simulink library "exprofilelib"  (Simulink 7.6)
settings: Solver=ode45  SolverMode=SingleTasking  StartTime=0.0  StopTime=10.0  RelTol=1e-3
undefined symbols (not defined in the file or in its folder): T
libraries: simulink x2, exprofilelib x1, simulink_extras x1
settings Model: Creator=The MathWorks Inc.

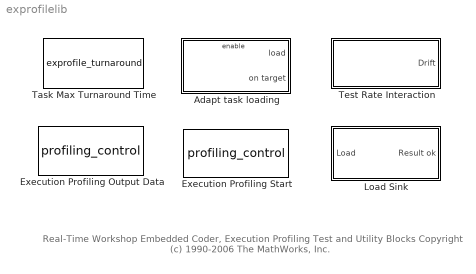
== system exprofilelib ==
  note: Real-Time Workshop Embedded Coder, Execution Profiling Test and Utility Blocks
      | Copyright (c) 1990-2006 The MathWorks, Inc.
  Adapt task loading : Subsystem  mask(Adapt task loading){rateNum=0, target=uint32(1000), adapt=64, t=T}
      mask prompts: rateNum "Rate number:"; target "Target turnaround time in free running timer ticks:"; adapt "Adaptation factor:"; t "Sample time:"
      mask help: Increase the load demand until the task turnaround time reaches the target. The load demand ratchets up at a rate inversely proportional to the adaptation factor.
      mask Display: disp(sprintf(['Target = %d'], double(target)))
  Execution Profiling Output Data : S-Function  FunctionName=profiling_control  Parameters=mode, t  EnableBusSupport=off  mask(Output execution profiling data){t=1}
      mask prompts: t "Sample time"
      mask help: Outputs logged exectution profiling data. The data is output 8 bytes at a time; the active output is set to true while logged data is output.
      mask init:
      | mode = 2; % data output
      mask Display:
      | port_label('output',1,'Data active')
      | port_label('output',2,'Data')
  Execution Profiling Start : S-Function  FunctionName=profiling_control  Parameters=mode, t  EnableBusSupport=off  mask(Start Execution Profiling){}
      mask help: Initiates logging of execution profiling data; this block should typically be placed inside a triggered sub-system.
      mask init:
      | mode = 1; % control input
      | t = -1; % sample time
      mask Display: disp(sprintf('Start\nExecution Profiling'))
  Load Sink : Subsystem  TreatAsAtomicUnit=on  mask(Load Sink){mode=single, t=1}
      mask prompts: t "Sample time:"
      mask help: This block consumes processor time by performing integer or floating point calculations. The larger the value of the load input, the more processor time is consumed.
      mask init:
      | if strcmp(mode,'int16')
      | 	tol_eps = int32(0);
      | 	a = int32(0);
      | elseif strcmp(mode,'single')
      |     tol_eps = single(1.192e-7);
      | 	a = single(3.1415926);
      | else
      | 	error(['Unrecognized value for mode'])
      | end
      settings: RTWSystemCode=Function
      mask StyleString: popup(int16|single),edit
  Task Max Turnaround Time : S-Function  FunctionName=exprofile_turnaround  Parameters=rateNumber, t  EnableBusSupport=off  mask(Task Maximum Turnaround Time){rateNumber=0, t=T*16}
      mask prompts: rateNumber "Rate number:"; t "Sample time:"
      mask help:
      | Outputs the maximum logged turnaround time, in free running timer ticks, for a model timer-based task. A free running timer must have been configured for use with the execution profiling engine. If execution profiling is not enabled, the output is zero.
      |
      | For a model running in multi-tasking mode, the rate number must be in the range 0 to (N-1) where 0 represents the base rate and N is the total number of rates in the model. If the model is running in single tasking mode then the rate number must be zero.
      mask Display: disp(sprintf('Task maximum\nturnaround time'))
  Test Rate Interaction : Subsystem  mask(Test Rate Interaction){t=T}
      mask prompts: t "Faster sample time:"
      mask help:
      | This block contains two tasks, one with the faster sample time, the other running four times slower.
      |
      | Data is transferred continually between the two tasks and tested for consistency. In simulation, the drift output will always be zero. When executing in real-time, the drift output will always be non-zero provided that no sub-rate overruns occur. If sub-rate overruns do occur then data transfer between rates may be delayed causing the drift output to be non-zero.
      mask Display: disp(sprintf('Test rate\n interaction'))

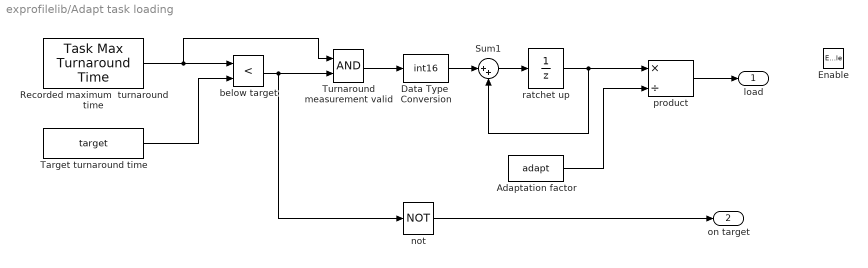
== system exprofilelib/Adapt task loading ==
  Enable : EnablePort
  Adaptation factor : Constant  Value=adapt  OutDataTypeStr=Inherit: Inherit via back propagation
  Data Type  Conversion : DataTypeConversion  OutDataTypeStr=int16  SaturateOnIntegerOverflow=on  RndMeth=Zero
  Recorded maximum  turnaround time : exprofilelib/Task Max Turnaround Time  rateNumber=rateNum  t=t
  Sum1 : Sum  Inputs=|++  InputSameDT=on
  Target turnaround time : Constant  Value=target
  Turnaround measurement valid : Logic  AllPortsSameDT=off  OutDataTypeStr=uint(8)
  below target : RelationalOperator  Operator=<  InputSameDT=on
  not : Logic  Operator=NOT  AllPortsSameDT=off  OutDataTypeStr=uint(8)
  product : Product  Inputs=*/  InputSameDT=on  OutDataTypeStr=Inherit: Same as first input
  ratchet up : UnitDelay  SampleTime=-1
  load : Outport
  on target : Outport  Port=2
  wires:
  not/1 -> on target/1
  Target turnaround time/1 -> below target/2
  product/1 -> load/1
  Recorded maximum  turnaround time/1 -> below target/1, Turnaround measurement valid/1
  Adaptation factor/1 -> product/2
  Data Type  Conversion/1 -> Sum1/1
  ratchet up/1 -> product/1, Sum1/2
  below target/1 -> not/1, Turnaround measurement valid/2
  Sum1/1 -> ratchet up/1
  Turnaround measurement valid/1 -> Data Type  Conversion/1

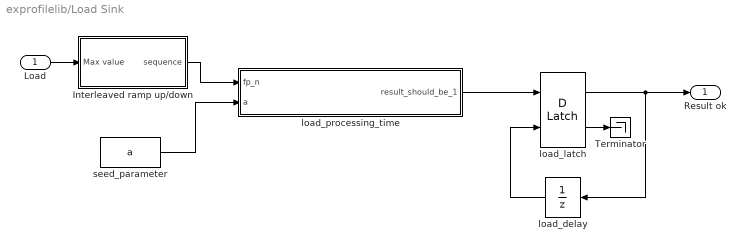
== system exprofilelib/Load Sink ==
  Load : Inport
  Interleaved ramp up/down : Subsystem  mask(Interleaved ramp up/down){t=t}
      mask prompts: t "Sample time:"
  Terminator : Terminator
  load_delay : UnitDelay  X0=1  SampleTime=t
  load_latch : simulink_extras/Flip Flops/D Latch  SystemSampleTime=-1
  load_processing_time : Subsystem
  seed_parameter : Constant  Value=a
  Result ok : Outport
  wires:
  seed_parameter/1 -> load_processing_time/2(a)
  load_processing_time/1(result_should_be_1) -> load_latch/1
  load_latch/1 -> Result ok/1, load_delay/1
  load_delay/1 -> load_latch/2
  load_latch/2 -> Terminator/1
  Interleaved ramp up/down/1(sequence) -> load_processing_time/1(fp_n)
  Load/1 -> Interleaved ramp up/down/1(Max value)

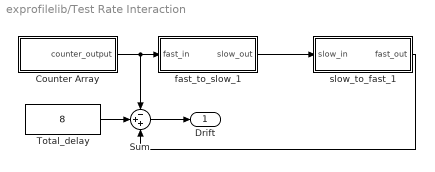
== system exprofilelib/Test Rate Interaction ==
  Counter Array : Subsystem
  Sum : Sum  Inputs=-++  InputSameDT=on
  Total_delay : Constant  Value=8  OutDataTypeStr=Inherit: Inherit via back propagation
  fast_to_slow_1 : Subsystem
  slow_to_fast_1 : Subsystem
  Drift : Outport
  wires:
  fast_to_slow_1/1(slow_out) -> slow_to_fast_1/1(slow_in)
  Counter Array/1(counter_output) -> fast_to_slow_1/1(fast_in), Sum/1
  Total_delay/1 -> Sum/2
  slow_to_fast_1/1(fast_out) -> Sum/3
  Sum/1 -> Drift/1

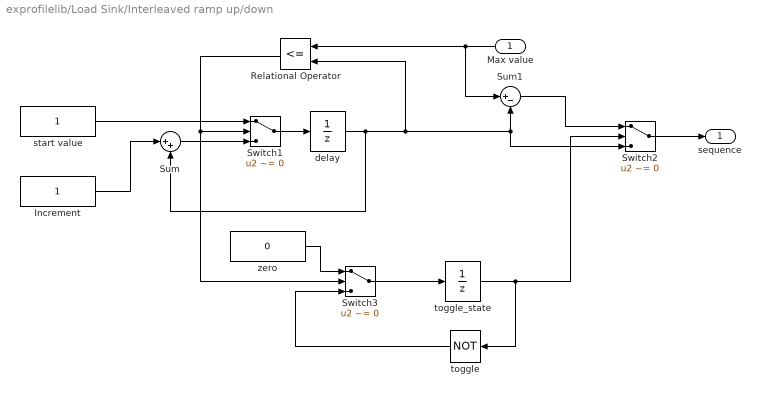
== system exprofilelib/Load Sink/Interleaved ramp up/down ==
  Max value : Inport
  Increment : Constant  OutDataTypeStr=Inherit: Inherit via back propagation
  Relational Operator : RelationalOperator  Operator=<=  InputSameDT=on
  Sum : Sum  Inputs=|++  InputSameDT=on
  Sum1 : Sum  Inputs=|+-
  Switch1 : Switch  Criteria=u2 ~= 0  SaturateOnIntegerOverflow=on  InputSameDT=on
  Switch2 : Switch  Criteria=u2 ~= 0  SaturateOnIntegerOverflow=on
  Switch3 : Switch  Criteria=u2 ~= 0  SaturateOnIntegerOverflow=on  InputSameDT=on
  delay : UnitDelay  X0=1  SampleTime=t
  start value : Constant  OutDataTypeStr=Inherit: Inherit via back propagation
  toggle : Logic  Operator=NOT  AllPortsSameDT=off
  toggle_state : UnitDelay  SampleTime=t
  zero : Constant  Value=0  OutDataTypeStr=Inherit: Inherit via back propagation
  sequence : Outport
  wires:
  zero/1 -> Switch3/1
  Switch3/1 -> toggle_state/1
  toggle/1 -> Switch3/3
  Sum1/1 -> Switch2/1
  toggle_state/1 -> Switch2/2, toggle/1
  start value/1 -> Switch1/1
  Switch2/1 -> sequence/1
  Max value/1 -> Sum1/1, Relational Operator/1
  Relational Operator/1 -> Switch3/2, Switch1/2
  Sum/1 -> Switch1/3
  Switch1/1 -> delay/1
  Increment/1 -> Sum/1
  delay/1 -> Switch2/3, Sum1/2, Relational Operator/2, Sum/2

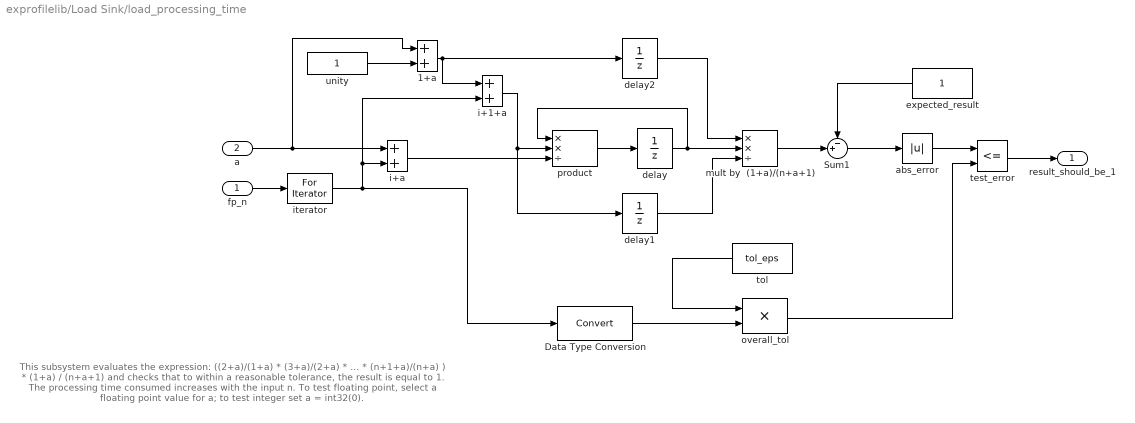
== system exprofilelib/Load Sink/load_processing_time ==
  note: This subsystem evaluates the expression:
      |
      | ((2+a)/(1+a) * (3+a)/(2+a) * ... * (n+1+a)/(n+a) ) * (1+a) / (n+a+1)
      |
      | and checks that to within a reasonable tolerance, the result is equal to 1.
      |
      | The processing time consumed increases with the input n. To test floating
      | point, select a floating point value for a; to test integer set a = int32(0).
  fp_n : Inport
  a : Inport  Port=2
  1+a : Sum  InputSameDT=on  OutDataTypeStr=Inherit: Same as first input
  Data Type Conversion : DataTypeConversion
  Sum1 : Sum  Inputs=-+|  InputSameDT=on
  abs_error : Abs  SaturateOnIntegerOverflow=on
  delay : UnitDelay  X0=1  SampleTime=-1
  delay1 : UnitDelay  X0=1  SampleTime=-1
  delay2 : UnitDelay  X0=1  SampleTime=-1
  expected_result : Constant  OutDataTypeStr=Inherit: Inherit via back propagation
  i+1+a : Sum  OutDataTypeStr=Inherit: Same as first input
  i+a : Sum  OutDataTypeStr=Inherit: Same as first input
  iterator : ForIterator  ResetStates=reset  IterationSource=external
  mult by  (1+a)/(n+a+1) : Product  Inputs=**/  OutDataTypeStr=Inherit: Same as first input
  overall_tol : Product  OutDataTypeStr=Inherit: Inherit via back propagation  InputSameDT=on
  product : Product  Inputs=**/  InputSameDT=on  OutDataTypeStr=Inherit: Same as first input
  test_error : RelationalOperator  Operator=<=  InputSameDT=on
  tol : Constant  Value=tol_eps
  unity : Constant  OutDataTypeStr=Inherit: Inherit via back propagation
  result_should_be_1 : Outport
  wires:
  delay2/1 -> mult by  (1+a)/(n+a+1)/1
  delay1/1 -> mult by  (1+a)/(n+a+1)/3
  i+1+a/1 -> delay1/1, product/2
  delay/1 -> mult by  (1+a)/(n+a+1)/2, product/1
  1+a/1 -> delay2/1, i+1+a/1
  i+a/1 -> product/3
  unity/1 -> 1+a/2
  a/1 -> 1+a/1, i+a/1
  iterator/1 -> i+1+a/2, i+a/2, Data Type Conversion/1
  test_error/1 -> result_should_be_1/1
  mult by  (1+a)/(n+a+1)/1 -> Sum1/2
  expected_result/1 -> Sum1/1
  Sum1/1 -> abs_error/1
  overall_tol/1 -> test_error/2
  abs_error/1 -> test_error/1
  tol/1 -> overall_tol/1
  product/1 -> delay/1
  fp_n/1 -> iterator/1
  Data Type Conversion/1 -> overall_tol/2

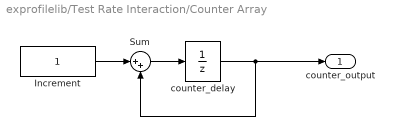
== system exprofilelib/Test Rate Interaction/Counter Array ==
  Increment : Constant  OutDataTypeStr=uint8
  Sum : Sum  Inputs=|++  InputSameDT=on
  counter_delay : UnitDelay  SampleTime=t
  counter_output : Outport
  wires:
  Sum/1 -> counter_delay/1
  counter_delay/1 -> Sum/2, counter_output/1
  Increment/1 -> Sum/1

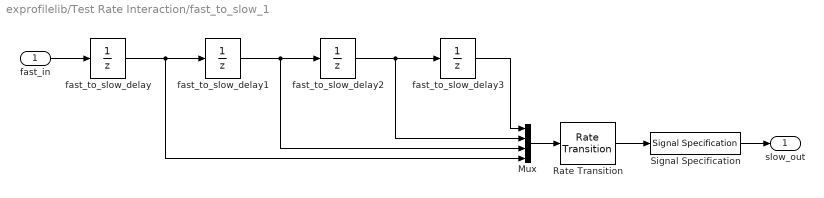
== system exprofilelib/Test Rate Interaction/fast_to_slow_1 ==
  fast_in : Inport
  Mux : Mux
  Rate Transition : simulink/Signal Attributes/Rate Transition  DataIntegrity=on  DeterministicTransfer=on  TransitionType=Fast to slow  InitCond=0
  Signal Specification : simulink/Signal Attributes/Signal Specification  D=-1  Ts=4*t  DataType=auto  OutDataType=sfix(16)  OutScaling=2^0
      settings: SignalType=auto  SamplingMode=auto
  fast_to_slow_delay : UnitDelay  X0=2^8 - 1  SampleTime=t
  fast_to_slow_delay1 : UnitDelay  X0=2^8 - 2  SampleTime=t
  fast_to_slow_delay2 : UnitDelay  X0=2^8 - 3  SampleTime=t
  fast_to_slow_delay3 : UnitDelay  X0=2^8 - 4  SampleTime=t
  slow_out : Outport
  wires:
  fast_in/1 -> fast_to_slow_delay/1
  Rate Transition/1 -> Signal Specification/1
  Mux/1 -> Rate Transition/1
  fast_to_slow_delay2/1 -> Mux/2, fast_to_slow_delay3/1
  fast_to_slow_delay1/1 -> fast_to_slow_delay2/1, Mux/3
  fast_to_slow_delay/1 -> fast_to_slow_delay1/1, Mux/4
  fast_to_slow_delay3/1 -> Mux/1
  Signal Specification/1 -> slow_out/1

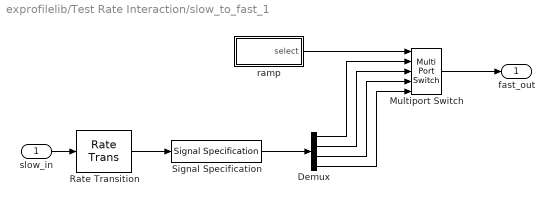
== system exprofilelib/Test Rate Interaction/slow_to_fast_1 ==
  slow_in : Inport
  Demux : Demux
  Multiport Switch : MultiPortSwitch  Inputs=4  zeroidx=off  SaturateOnIntegerOverflow=on
  Rate Transition : RateTransition  X0=[2^8*ones(1,4) - [8 7 6 5] ]
  Signal Specification : SignalSpecification  SampleTime=t
  ramp : Subsystem
  fast_out : Outport
  wires:
  Multiport Switch/1 -> fast_out/1
  Demux/4 -> Multiport Switch/5
  Demux/3 -> Multiport Switch/4
  Demux/2 -> Multiport Switch/3
  Demux/1 -> Multiport Switch/2
  Signal Specification/1 -> Demux/1
  ramp/1(select) -> Multiport Switch/1
  Rate Transition/1 -> Signal Specification/1
  slow_in/1 -> Rate Transition/1

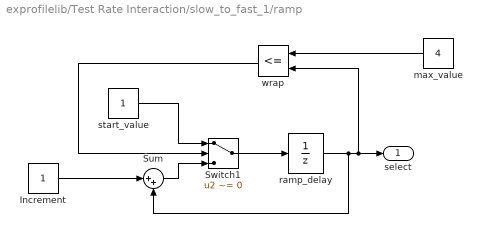
== system exprofilelib/Test Rate Interaction/slow_to_fast_1/ramp ==
  Increment : Constant  OutDataTypeStr=uint8
  Sum : Sum  Inputs=|++  SaturateOnIntegerOverflow=on  InputSameDT=on
  Switch1 : Switch  Criteria=u2 ~= 0  SaturateOnIntegerOverflow=on
  max_value : Constant  Value=4  OutDataTypeStr=uint8
  ramp_delay : UnitDelay  X0=1  SampleTime=t
  start_value : Constant  OutDataTypeStr=uint8
  wrap : RelationalOperator  Operator=<=
  select : Outport
  wires:
  Sum/1 -> Switch1/3
  Increment/1 -> Sum/1
  start_value/1 -> Switch1/1
  wrap/1 -> Switch1/2
  max_value/1 -> wrap/1
  ramp_delay/1 -> Sum/2, wrap/2, select/1
  Switch1/1 -> ramp_delay/1
